simulink model "DYNctl_ver4_etud_Avec_AsservissementNONfonctionnel"  (R2021b)
settings: Solver=ode45  StartTime=0.0  StopTime=tfin  FixedStep=0.001  RelTol=1e-09  EnableMultiTasking=on
values from neighbouring files (symbols this model uses):
  A = num_pos_sph(3)    [Compensateur.m]    (also in matrice_L.m = sym(zeros(13, 13)))
  ae0 = 0.000013398315537 * 1.0e+5    (= 1.3398315537)    [bancEssaiConstantes.m]
  ae1 = 0.003556457401249 * 1.0e+5    (= 355.645740125)    [bancEssaiConstantes.m]
  ae2 = 0.018168930792891 * 1.0e+5    (= 1816.89307929)    [bancEssaiConstantes.m]
  ae3 = 7.043847497815494 * 1.0e+5    (= 704384.749782)    [bancEssaiConstantes.m]
  as0 = 0.0609    [bancEssaiConstantes.m]
  as1 = 18.1233    [bancEssaiConstantes.m]
  as2 = 3.1142e+03    (= 3114.2)    [bancEssaiConstantes.m]
  as3 = -2.3281e+05    (= -232810)    [bancEssaiConstantes.m]
  Axeq = 0    [run_bancessai.m]
  Ayeq = 0    [run_bancessai.m]
  B = [B1 ... (first row only)    [matrice_L.m]
  be1 = 13.029359254409743    (= 13.0293592544)    [bancEssaiConstantes.m]
  C = [Tdef C3 C3 C3 C2 ... (first row only)    [matrice_L.m]
  D = [sum(distance);sum(distance.*voltage)]    [Capteur.m]    (also in matrice_L.m = [0])
  g = 9.81    [bancEssaiConstantes.m]    (also in courant_voltage.m; matrice_L.m; projet.m; trajectoire.m = sqrt(1+(yd).^2))
  Jy = Jx    (= 0.001169)    [bancEssaiConstantes.m]    (also in courant_voltage.m = 0.001347; matrice_L.m = 0.001347)
  Kp_pos_sph = (wn_pos_sph^2)/A_pos_sph    [Compensateur_position_sphere.m]
  Kv_pos_sph = (2*zeta_pos_sph*wn_pos_sph)/A_pos_sph    [Compensateur_position_sphere.m]
  LA = LL    (= 0.115)    [bancEssaiConstantes.m]
  LB = LL    (= 0.115)    [bancEssaiConstantes.m]
  LC = LL    (= 0.115)    [bancEssaiConstantes.m]
  mS = 0.0080    (= 0.008)    [bancEssaiConstantes.m]
  mtot = mP + sig*mS    [bancEssaiConstantes.m]
  Px_eq_simu = double(Px_eq)    [matrice_L.m]
  Py_eq_simu = double(Py_eq)    [matrice_L.m]
  Pzeq = .015    (= 0.015)    [run_bancessai.m]
  RA = RR    (= 3.6)    [bancEssaiConstantes.m]
  RB = RR    (= 3.6)    [bancEssaiConstantes.m]
  RC = RR    (= 3.6)    [bancEssaiConstantes.m]
  TABC_inv = inv(TABC)    [bancEssaiConstantes.m]
  TDEF_inv = inv(TDEF)    [bancEssaiConstantes.m]
  Uinv = inv(U)    [matrice_L.m]
  Va_eq_simu = double(Va_eq)    [courant_voltage.m]
  Vb_eq_simu = double(Vb_eq)    [courant_voltage.m]
  Vc_eq_simu = double(Vc_eq)    [courant_voltage.m]
  Vmax = 22.0    (= 22)    [bancEssaiConstantes.m]
  XB = -rABC*sind(30)    [bancEssaiConstantes.m]    (also in courant_voltage.m = - XA*sind(30); matrice_L.m = -XA*sind(30); projet.m = XA*sind(30))
  XC = -rABC*sind(30)    [bancEssaiConstantes.m]    (also in courant_voltage.m = - XA*sind(30); matrice_L.m = -XA*sind(30); projet.m = XA*sind(30))
  YB = +rABC*cosd(30)    [bancEssaiConstantes.m]    (also in courant_voltage.m = XA*cosd(30); matrice_L.m = XA*cosd(30))
  YC = -rABC*cosd(30)    [bancEssaiConstantes.m]    (also in courant_voltage.m = -XA*cosd(30); matrice_L.m = -XA*cosd(30))
undefined symbols (not defined in the file or in its folder): A_phi, A_s, A_theta, A_z, B_phi, B_sx, B_sy, B_theta, B_z, C_dec, C_s, D_dec, D_s, den_hpc2, den_ip, num_hpc2, num_ip, Tdeft, Tdeft2, U_U_simu
(part 2 of 2)

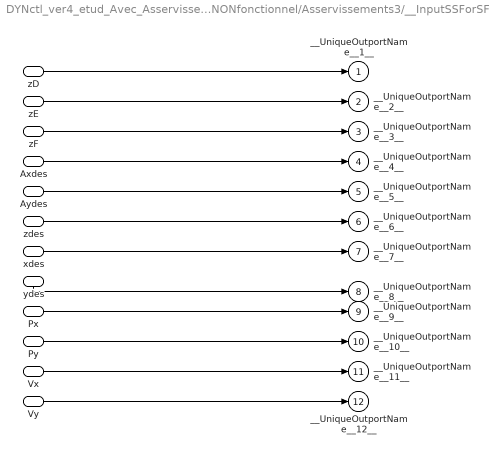
== system DYNctl_ver4_etud_Avec_AsservissementNONfonctionnel/Asservissements3/__InputSSForSFun__ ==
  zD : Inport
  zE : Inport  Port=2
  zF : Inport  Port=3
  Axdes : Inport  Port=4
  Aydes : Inport  Port=5
  zdes : Inport  Port=6
  xdes : Inport  Port=7
  ydes : Inport  Port=8
  Px : Inport  Port=9
  Py : Inport  Port=10
  Vx : Inport  Port=11
  Vy : Inport  Port=12
  __UniqueOutportName__1__ : Outport  VectorParamsAs1DForOutWhenUnconnected=off
  __UniqueOutportName__2__ : Outport  Port=2  VectorParamsAs1DForOutWhenUnconnected=off
  __UniqueOutportName__3__ : Outport  Port=3  VectorParamsAs1DForOutWhenUnconnected=off
  __UniqueOutportName__4__ : Outport  Port=4  VectorParamsAs1DForOutWhenUnconnected=off
  __UniqueOutportName__5__ : Outport  Port=5  VectorParamsAs1DForOutWhenUnconnected=off
  __UniqueOutportName__6__ : Outport  Port=6  VectorParamsAs1DForOutWhenUnconnected=off
  __UniqueOutportName__7__ : Outport  Port=7  VectorParamsAs1DForOutWhenUnconnected=off
  __UniqueOutportName__8__ : Outport  Port=8  VectorParamsAs1DForOutWhenUnconnected=off
  __UniqueOutportName__9__ : Outport  Port=9  VectorParamsAs1DForOutWhenUnconnected=off
  __UniqueOutportName__10__ : Outport  Port=10  VectorParamsAs1DForOutWhenUnconnected=off
  __UniqueOutportName__11__ : Outport  Port=11  VectorParamsAs1DForOutWhenUnconnected=off
  __UniqueOutportName__12__ : Outport  Port=12  VectorParamsAs1DForOutWhenUnconnected=off
  wires:
  zD/1 -> __UniqueOutportName__1__/1
  zE/1 -> __UniqueOutportName__2__/1
  zF/1 -> __UniqueOutportName__3__/1
  Axdes/1 -> __UniqueOutportName__4__/1
  Aydes/1 -> __UniqueOutportName__5__/1
  zdes/1 -> __UniqueOutportName__6__/1
  xdes/1 -> __UniqueOutportName__7__/1
  ydes/1 -> __UniqueOutportName__8__/1
  Px/1 -> __UniqueOutportName__9__/1
  Py/1 -> __UniqueOutportName__10__/1
  Vx/1 -> __UniqueOutportName__11__/1
  Vy/1 -> __UniqueOutportName__12__/1

== system DYNctl_ver4_etud_Avec_AsservissementNONfonctionnel/Asservissements3/__OutputSSForSFun__ ==
  __UniqueInportName__1__ : Inport
  __UniqueInportName__2__ : Inport  Port=2
  __UniqueInportName__3__ : Inport  Port=3
  __UniqueInportName__4__ : Inport  Port=4
  __UniqueInportName__5__ : Inport  Port=5
  VAcalcule : Outport  VectorParamsAs1DForOutWhenUnconnected=off
  VBcalcule : Outport  Port=2  VectorParamsAs1DForOutWhenUnconnected=off
  VCcalcule : Outport  Port=3  VectorParamsAs1DForOutWhenUnconnected=off
  Axcalcule : Outport  Port=4  VectorParamsAs1DForOutWhenUnconnected=off
  Aycalcule : Outport  Port=5  VectorParamsAs1DForOutWhenUnconnected=off
  wires:
  __UniqueInportName__1__/1 -> VAcalcule/1
  __UniqueInportName__2__/1 -> VBcalcule/1
  __UniqueInportName__3__/1 -> VCcalcule/1
  __UniqueInportName__4__/1 -> Axcalcule/1  "Ax_des"
  __UniqueInportName__5__/1 -> Aycalcule/1  "Ay_des"

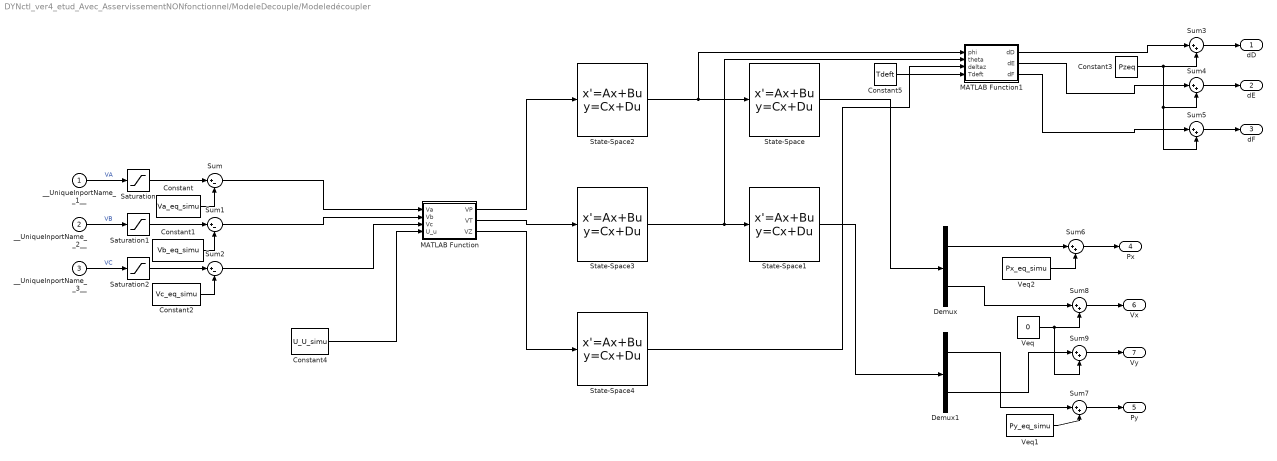
== system DYNctl_ver4_etud_Avec_AsservissementNONfonctionnel/ModeleDecouple/Modeledécoupler ==
  __UniqueInportName__1__ : Inport
  __UniqueInportName__2__ : Inport  Port=2
  __UniqueInportName__3__ : Inport  Port=3
  Constant : Constant  Value=Va_eq_simu
  Constant1 : Constant  Value=Vb_eq_simu
  Constant2 : Constant  Value=Vc_eq_simu
  Constant3 : Constant  Value=Pzeq
  Constant4 : Constant  Value=U_U_simu
  Constant5 : Constant  Value=Tdeft
  Demux : Demux  Outputs=2
  Demux1 : Demux  Outputs=2
  MATLAB Function : MATLAB Function  TreatAsAtomicUnit=on
  MATLAB Function1 : MATLAB Function  TreatAsAtomicUnit=on
  Saturation : Saturate  UpperLimit=Vmax  LowerLimit=-Vmax
  Saturation1 : Saturate  UpperLimit=Vmax  LowerLimit=-Vmax
  Saturation2 : Saturate  UpperLimit=Vmax  LowerLimit=-Vmax
  State-Space : StateSpace  A=A_s  B=B_sx  C=C_s  D=D_s  InitialCondition=0
  State-Space1 : StateSpace  A=A_s  B=B_sy  C=C_s  D=D_s  InitialCondition=0
  State-Space2 : StateSpace  A=A_phi  B=B_phi  C=C_dec  D=D_dec  InitialCondition=0
  State-Space3 : StateSpace  A=A_theta  B=B_theta  C=C_dec  D=D_dec  InitialCondition=0
  State-Space4 : StateSpace  A=A_z  B=B_z  C=C_dec  D=D_dec  InitialCondition=0
  Sum : Sum  Inputs=|+-
  Sum1 : Sum  Inputs=|+-
  Sum2 : Sum  Inputs=|+-
  Sum{3..9} (7 alike) : Sum  Inputs=|++
  Veq : Constant  Value=0  VectorParams1D=off
  Veq1 : Constant  Value=Py_eq_simu
  Veq2 : Constant  Value=Px_eq_simu
  dD : Outport  VectorParamsAs1DForOutWhenUnconnected=off
  dE : Outport  Port=2  VectorParamsAs1DForOutWhenUnconnected=off
  dF : Outport  Port=3  VectorParamsAs1DForOutWhenUnconnected=off
  Px : Outport  Port=4  VectorParamsAs1DForOutWhenUnconnected=off
  Py : Outport  Port=5  VectorParamsAs1DForOutWhenUnconnected=off
  Vx : Outport  Port=6  VectorParamsAs1DForOutWhenUnconnected=off
  Vy : Outport  Port=7  VectorParamsAs1DForOutWhenUnconnected=off
  wires:
  __UniqueInportName__1__/1 -> Saturation/1  "VA"
  __UniqueInportName__2__/1 -> Saturation1/1  "VB"
  __UniqueInportName__3__/1 -> Saturation2/1  "VC"
  Constant/1 -> Sum/2
  Sum/1 -> MATLAB Function/1(Va)
  Constant1/1 -> Sum1/2
  Sum1/1 -> MATLAB Function/2(Vb)
  Constant2/1 -> Sum2/2
  Sum2/1 -> MATLAB Function/3(Vc)
  Sum6/1 -> Px/1
  Sum7/1 -> Py/1
  Sum8/1 -> Vx/1
  Sum9/1 -> Vy/1
  Veq/1 -> Sum8/2, Sum9/2
  Veq1/1 -> Sum7/2
  Veq2/1 -> Sum6/2
  Sum3/1 -> dD/1
  Saturation/1 -> Sum/1
  Saturation1/1 -> Sum1/1
  Saturation2/1 -> Sum2/1
  State-Space3/1 -> MATLAB Function1/2(theta), State-Space1/1
  State-Space2/1 -> MATLAB Function1/1(phi), State-Space/1
  Constant4/1 -> MATLAB Function/4(U_u)
  MATLAB Function/1(VP) -> State-Space2/1
  MATLAB Function/2(VT) -> State-Space3/1
  MATLAB Function/3(VZ) -> State-Space4/1
  State-Space/1 -> Demux/1
  State-Space1/1 -> Demux1/1
  Constant3/1 -> Sum4/2, Sum5/2, Sum3/2
  Sum5/1 -> dF/1
  Sum4/1 -> dE/1
  State-Space4/1 -> MATLAB Function1/3(deltaz)
  Constant5/1 -> MATLAB Function1/4(Tdeft)
  MATLAB Function1/1(dD) -> Sum3/1
  MATLAB Function1/2(dE) -> Sum4/1
  MATLAB Function1/3(dF) -> Sum5/1
  Demux/1 -> Sum6/1
  Demux/2 -> Sum8/1
  Demux1/1 -> Sum7/1
  Demux1/2 -> Sum9/1

== system DYNctl_ver4_etud_Avec_AsservissementNONfonctionnel/ModeleDecouple/__InputSSForSFun__ ==
  VAdesire : Inport
  VBdesire : Inport  Port=2
  VCdesire : Inport  Port=3
  __UniqueOutportName__1__ : Outport  VectorParamsAs1DForOutWhenUnconnected=off
  __UniqueOutportName__2__ : Outport  Port=2  VectorParamsAs1DForOutWhenUnconnected=off
  __UniqueOutportName__3__ : Outport  Port=3  VectorParamsAs1DForOutWhenUnconnected=off
  wires:
  VAdesire/1 -> __UniqueOutportName__1__/1
  VBdesire/1 -> __UniqueOutportName__2__/1
  VCdesire/1 -> __UniqueOutportName__3__/1

== system DYNctl_ver4_etud_Avec_AsservissementNONfonctionnel/ModeleDecouple/__OutputSSForSFun__ ==
  __UniqueInportName__17__1 : Inport
  __UniqueInportName__18__ : Inport  Port=2
  __UniqueInportName__19__ : Inport  Port=3
  __UniqueInportName__7__ : Inport  Port=4
  __UniqueInportName__8__ : Inport  Port=5
  __UniqueInportName__9__ : Inport  Port=6
  __UniqueInportName__10__ : Inport  Port=7
  zD1 : Outport  VectorParamsAs1DForOutWhenUnconnected=off
  zE1 : Outport  Port=2  VectorParamsAs1DForOutWhenUnconnected=off
  zF1 : Outport  Port=3  VectorParamsAs1DForOutWhenUnconnected=off
  Px : Outport  Port=4  VectorParamsAs1DForOutWhenUnconnected=off
  Py : Outport  Port=5  VectorParamsAs1DForOutWhenUnconnected=off
  Vx : Outport  Port=6  VectorParamsAs1DForOutWhenUnconnected=off
  Vy : Outport  Port=7  VectorParamsAs1DForOutWhenUnconnected=off
  wires:
  __UniqueInportName__19__/1 -> zF1/1  "zf"
  __UniqueInportName__18__/1 -> zE1/1  "ze"
  __UniqueInportName__17__1/1 -> zD1/1  "zd"
  __UniqueInportName__10__/1 -> Vy/1  "Vy"
  __UniqueInportName__9__/1 -> Vx/1  "Vx"
  __UniqueInportName__8__/1 -> Py/1  "Py"
  __UniqueInportName__7__/1 -> Px/1  "Px"

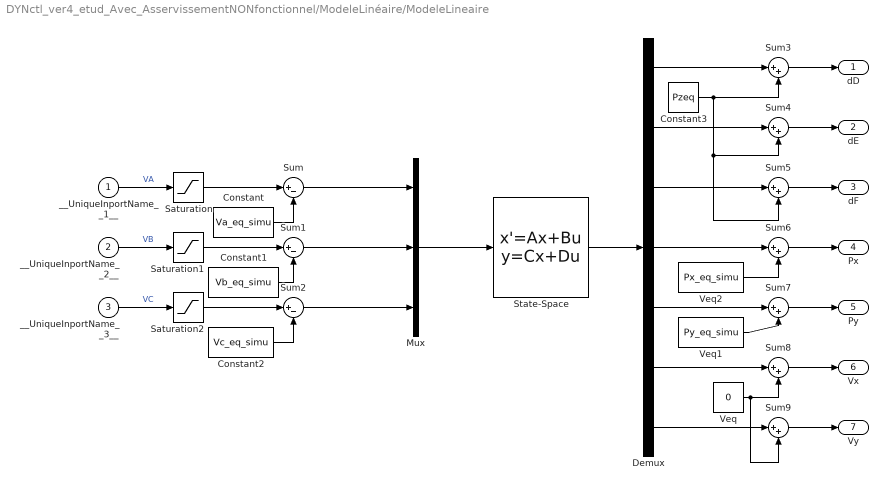
== system DYNctl_ver4_etud_Avec_AsservissementNONfonctionnel/ModeleLinéaire/ModeleLineaire ==
  __UniqueInportName__1__ : Inport
  __UniqueInportName__2__ : Inport  Port=2
  __UniqueInportName__3__ : Inport  Port=3
  Constant : Constant  Value=Va_eq_simu
  Constant1 : Constant  Value=Vb_eq_simu
  Constant2 : Constant  Value=Vc_eq_simu
  Constant3 : Constant  Value=Pzeq
  Demux : Demux  Outputs=7
  Mux : Mux  Inputs=3
  Saturation : Saturate  UpperLimit=Vmax  LowerLimit=-Vmax
  Saturation1 : Saturate  UpperLimit=Vmax  LowerLimit=-Vmax
  Saturation2 : Saturate  UpperLimit=Vmax  LowerLimit=-Vmax
  State-Space : StateSpace  A=A  B=B  C=C  D=D  InitialCondition=0
  Sum : Sum  Inputs=|+-
  Sum1 : Sum  Inputs=|+-
  Sum2 : Sum  Inputs=|+-
  Sum{3..9} (7 alike) : Sum  Inputs=|++
  Veq : Constant  Value=0
  Veq1 : Constant  Value=Py_eq_simu
  Veq2 : Constant  Value=Px_eq_simu
  dD : Outport  VectorParamsAs1DForOutWhenUnconnected=off
  dE : Outport  Port=2  VectorParamsAs1DForOutWhenUnconnected=off
  dF : Outport  Port=3  VectorParamsAs1DForOutWhenUnconnected=off
  Px : Outport  Port=4  VectorParamsAs1DForOutWhenUnconnected=off
  Py : Outport  Port=5  VectorParamsAs1DForOutWhenUnconnected=off
  Vx : Outport  Port=6  VectorParamsAs1DForOutWhenUnconnected=off
  Vy : Outport  Port=7  VectorParamsAs1DForOutWhenUnconnected=off
  wires:
  __UniqueInportName__1__/1 -> Saturation/1  "VA"
  __UniqueInportName__2__/1 -> Saturation1/1  "VB"
  __UniqueInportName__3__/1 -> Saturation2/1  "VC"
  Mux/1 -> State-Space/1
  State-Space/1 -> Demux/1
  Constant/1 -> Sum/2
  Sum/1 -> Mux/1
  Constant1/1 -> Sum1/2
  Sum1/1 -> Mux/2
  Constant2/1 -> Sum2/2
  Sum2/1 -> Mux/3
  Sum6/1 -> Px/1
  Sum7/1 -> Py/1
  Sum8/1 -> Vx/1
  Sum9/1 -> Vy/1
  Veq/1 -> Sum9/2, Sum8/2
  Demux/7 -> Sum9/1
  Demux/6 -> Sum8/1
  Veq1/1 -> Sum7/2
  Demux/5 -> Sum7/1
  Veq2/1 -> Sum6/2
  Demux/4 -> Sum6/1
  Constant3/1 -> Sum3/2, Sum4/2, Sum5/2
  Demux/1 -> Sum3/1
  Demux/2 -> Sum4/1
  Demux/3 -> Sum5/1
  Sum5/1 -> dF/1
  Sum3/1 -> dD/1
  Sum4/1 -> dE/1
  Saturation/1 -> Sum/1
  Saturation1/1 -> Sum1/1
  Saturation2/1 -> Sum2/1

== system DYNctl_ver4_etud_Avec_AsservissementNONfonctionnel/ModeleLinéaire/__InputSSForSFun__ ==
  VAdesire : Inport
  VBdesire : Inport  Port=2
  VCdesire : Inport  Port=3
  __UniqueOutportName__1__ : Outport  VectorParamsAs1DForOutWhenUnconnected=off
  __UniqueOutportName__2__ : Outport  Port=2  VectorParamsAs1DForOutWhenUnconnected=off
  __UniqueOutportName__3__ : Outport  Port=3  VectorParamsAs1DForOutWhenUnconnected=off
  wires:
  VAdesire/1 -> __UniqueOutportName__1__/1
  VBdesire/1 -> __UniqueOutportName__2__/1
  VCdesire/1 -> __UniqueOutportName__3__/1

== system DYNctl_ver4_etud_Avec_AsservissementNONfonctionnel/ModeleLinéaire/__OutputSSForSFun__ ==
  __UniqueInportName__17__ : Inport
  __UniqueInportName__18__ : Inport  Port=2
  __UniqueInportName__19__ : Inport  Port=3
  __UniqueInportName__7__ : Inport  Port=4
  __UniqueInportName__8__ : Inport  Port=5
  __UniqueInportName__9__ : Inport  Port=6
  __UniqueInportName__10__ : Inport  Port=7
  zD : Outport  VectorParamsAs1DForOutWhenUnconnected=off
  zE : Outport  Port=2  VectorParamsAs1DForOutWhenUnconnected=off
  zF : Outport  Port=3  VectorParamsAs1DForOutWhenUnconnected=off
  Px : Outport  Port=4  VectorParamsAs1DForOutWhenUnconnected=off
  Py : Outport  Port=5  VectorParamsAs1DForOutWhenUnconnected=off
  Vx : Outport  Port=6  VectorParamsAs1DForOutWhenUnconnected=off
  Vy : Outport  Port=7  VectorParamsAs1DForOutWhenUnconnected=off
  wires:
  __UniqueInportName__7__/1 -> Px/1  "Px"
  __UniqueInportName__8__/1 -> Py/1  "Py"
  __UniqueInportName__9__/1 -> Vx/1  "Vx"
  __UniqueInportName__10__/1 -> Vy/1  "Vy"
  __UniqueInportName__17__/1 -> zD/1  "zd"
  __UniqueInportName__18__/1 -> zE/1  "ze"
  __UniqueInportName__19__/1 -> zF/1  "zf"

== system DYNctl_ver4_etud_Avec_AsservissementNONfonctionnel/ModeleNonLineaire/__InputSSForSFun__ ==
  VAdesire : Inport
  VBdesire : Inport  Port=2
  VCdesire : Inport  Port=3
  __UniqueOutportName__1__ : Outport
  __UniqueOutportName__2__ : Outport  Port=2
  __UniqueOutportName__3__ : Outport  Port=3
  wires:
  VAdesire/1 -> __UniqueOutportName__1__/1
  VBdesire/1 -> __UniqueOutportName__2__/1
  VCdesire/1 -> __UniqueOutportName__3__/1

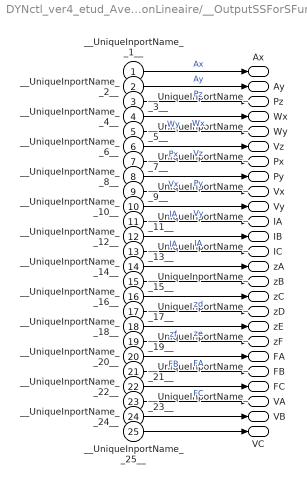
== system DYNctl_ver4_etud_Avec_AsservissementNONfonctionnel/ModeleNonLineaire/__OutputSSForSFun__ ==
  __UniqueInportName__1__ : Inport
  __UniqueInportName__2__ : Inport  Port=2
  __UniqueInportName__3__ : Inport  Port=3
  __UniqueInportName__4__ : Inport  Port=4
  __UniqueInportName__5__ : Inport  Port=5
  __UniqueInportName__6__ : Inport  Port=6
  __UniqueInportName__7__ : Inport  Port=7
  __UniqueInportName__8__ : Inport  Port=8
  __UniqueInportName__9__ : Inport  Port=9
  __UniqueInportName__10__ : Inport  Port=10
  __UniqueInportName__11__ : Inport  Port=11
  __UniqueInportName__12__ : Inport  Port=12
  __UniqueInportName__13__ : Inport  Port=13
  __UniqueInportName__14__ : Inport  Port=14
  __UniqueInportName__15__ : Inport  Port=15
  __UniqueInportName__16__ : Inport  Port=16
  __UniqueInportName__17__ : Inport  Port=17
  __UniqueInportName__18__ : Inport  Port=18
  __UniqueInportName__19__ : Inport  Port=19
  __UniqueInportName__20__ : Inport  Port=20
  __UniqueInportName__21__ : Inport  Port=21
  __UniqueInportName__22__ : Inport  Port=22
  __UniqueInportName__23__ : Inport  Port=23
  __UniqueInportName__24__ : Inport  Port=24
  __UniqueInportName__25__ : Inport  Port=25
  Ax : Outport
  Ay : Outport  Port=2
  Pz : Outport  Port=3
  Wx : Outport  Port=4
  Wy : Outport  Port=5
  Vz : Outport  Port=6
  Px : Outport  Port=7
  Py : Outport  Port=8
  Vx : Outport  Port=9
  Vy : Outport  Port=10
  IA : Outport  Port=11
  IB : Outport  Port=12
  IC : Outport  Port=13
  zA : Outport  Port=14
  zB : Outport  Port=15
  zC : Outport  Port=16
  zD : Outport  Port=17
  zE : Outport  Port=18
  zF : Outport  Port=19
  FA : Outport  Port=20
  FB : Outport  Port=21
  FC : Outport  Port=22
  VA : Outport  Port=23
  VB : Outport  Port=24
  VC : Outport  Port=25
  wires:
  __UniqueInportName__1__/1 -> Ax/1  "Ax"
  __UniqueInportName__2__/1 -> Ay/1  "Ay"
  __UniqueInportName__3__/1 -> Pz/1  "Pz"
  __UniqueInportName__4__/1 -> Wx/1  "Wx"
  __UniqueInportName__5__/1 -> Wy/1  "Wy"
  __UniqueInportName__6__/1 -> Vz/1  "Vz"
  __UniqueInportName__7__/1 -> Px/1  "Px"
  __UniqueInportName__8__/1 -> Py/1  "Py"
  __UniqueInportName__9__/1 -> Vx/1  "Vx"
  __UniqueInportName__10__/1 -> Vy/1  "Vy"
  __UniqueInportName__11__/1 -> IA/1  "IA"
  __UniqueInportName__12__/1 -> IB/1  "IA"
  __UniqueInportName__13__/1 -> IC/1  "IA"
  __UniqueInportName__14__/1 -> zA/1
  __UniqueInportName__15__/1 -> zB/1
  __UniqueInportName__16__/1 -> zC/1
  __UniqueInportName__17__/1 -> zD/1  "zd"
  __UniqueInportName__18__/1 -> zE/1  "ze"
  __UniqueInportName__19__/1 -> zF/1  "zf"
  __UniqueInportName__20__/1 -> FA/1  "FA"
  __UniqueInportName__21__/1 -> FB/1  "FB"
  __UniqueInportName__22__/1 -> FC/1  "FC"
  __UniqueInportName__23__/1 -> VA/1
  __UniqueInportName__24__/1 -> VB/1
  __UniqueInportName__25__/1 -> VC/1

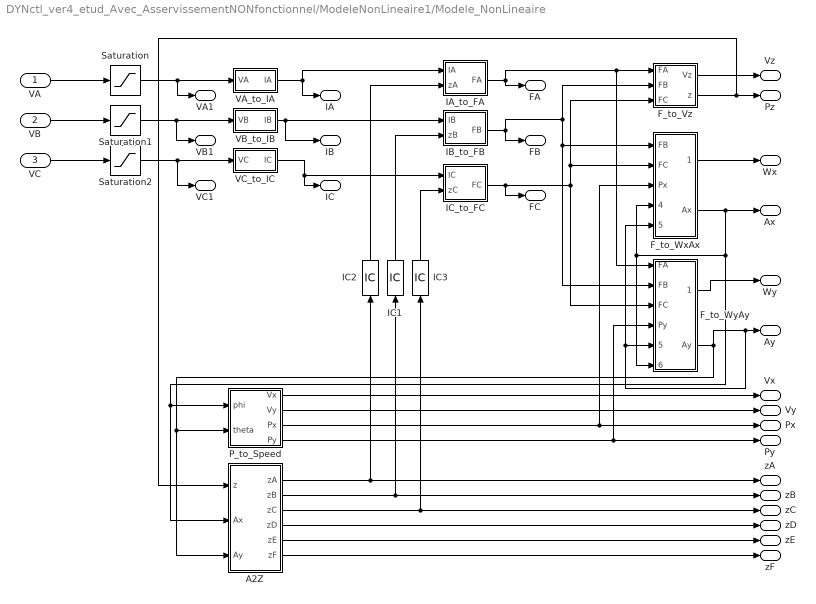
== system DYNctl_ver4_etud_Avec_AsservissementNONfonctionnel/ModeleNonLineaire1/Modele_NonLineaire ==
  VA : Inport
  VB : Inport  Port=2
  VC : Inport  Port=3
  A2Z : Subsystem
  F_to_Vz : Subsystem
  F_to_WxAx : Subsystem
  F_to_WyAy : Subsystem
  IA_to_FA : Subsystem
  IB_to_FB : Subsystem
  IC1 : InitialCondition  Value=Pzeq
  IC2 : InitialCondition  Value=Pzeq
  IC3 : InitialCondition  Value=Pzeq
  IC_to_FC : Subsystem
  P_to_Speed : Subsystem
  Saturation : Saturate  UpperLimit=Vmax  LowerLimit=-Vmax
  Saturation1 : Saturate  UpperLimit=Vmax  LowerLimit=-Vmax
  Saturation2 : Saturate  UpperLimit=Vmax  LowerLimit=-Vmax
  VA_to_IA : Subsystem
  VB_to_IB : Subsystem
  VC_to_IC : Subsystem
  Ax : Outport
  Ay : Outport  Port=2
  Pz : Outport  Port=3
  Wx : Outport  Port=4
  Wy : Outport  Port=5
  Vz : Outport  Port=6
  Px : Outport  Port=7
  Py : Outport  Port=8
  Vx : Outport  Port=9
  Vy : Outport  Port=10
  IA : Outport  Port=11
  IB : Outport  Port=12
  IC : Outport  Port=13
  zA : Outport  Port=14
  zB : Outport  Port=15
  zC : Outport  Port=16
  zD : Outport  Port=17
  zE : Outport  Port=18
  zF : Outport  Port=19
  FA : Outport  Port=20
  FB : Outport  Port=21
  FC : Outport  Port=22
  VA1 : Outport  Port=23
  VB1 : Outport  Port=24
  VC1 : Outport  Port=25
  wires:
  VA/1 -> Saturation/1
  VB/1 -> Saturation1/1
  VC/1 -> Saturation2/1
  VA_to_IA/1(IA) -> IA/1, IA_to_FA/1(IA)
  VB_to_IB/1(IB) -> IB/1, IB_to_FB/1(IB)
  VC_to_IC/1(IC) -> IC_to_FC/1(IC), IC/1
  IC_to_FC/1(FC) -> F_to_WyAy/3(FC), F_to_WxAx/2(FC), F_to_Vz/3(FC), FC/1
  IB_to_FB/1(FB) -> F_to_WyAy/2(FB), F_to_WxAx/1(FB), F_to_Vz/2(FB), FB/1
  IA_to_FA/1(FA) -> F_to_WyAy/1(FA), F_to_Vz/1(FA), FA/1
  F_to_WxAx/2(Ax) -> P_to_Speed/1(phi), A2Z/2(Ax), F_to_WyAy/6(phi), F_to_WxAx/4(phi), Ax/1
  F_to_WyAy/2(Ay) -> F_to_WxAx/5(theta), F_to_WyAy/5(theta), Ay/1, P_to_Speed/2(theta), A2Z/3(Ay)
  F_to_WyAy/1(Wy) -> Wy/1
  F_to_Vz/1(Vz) -> Vz/1
  F_to_WxAx/1(Wx) -> Wx/1
  P_to_Speed/1(Vx) -> Vx/1
  P_to_Speed/2(Vy) -> Vy/1
  F_to_Vz/2(z) -> A2Z/1(z), Pz/1
  P_to_Speed/3(Px) -> Px/1, F_to_WxAx/3(Px)
  P_to_Speed/4(Py) -> Py/1, F_to_WyAy/4(Py)
  A2Z/6(zF) -> zF/1
  A2Z/1(zA) -> zA/1, IC2/1
  A2Z/5(zE) -> zE/1
  A2Z/2(zB) -> zB/1, IC1/1
  A2Z/3(zC) -> zC/1, IC3/1
  A2Z/4(zD) -> zD/1
  Saturation/1 -> VA1/1, VA_to_IA/1(VA)
  Saturation1/1 -> VB1/1, VB_to_IB/1(VB)
  Saturation2/1 -> VC1/1, VC_to_IC/1(VC)
  IC2/1 -> IA_to_FA/2(zA)
  IC1/1 -> IB_to_FB/2(zB)
  IC3/1 -> IC_to_FC/2(zC)

== system DYNctl_ver4_etud_Avec_AsservissementNONfonctionnel/ModeleNonLineaire1/__InputSSForSFun__ ==
  VAdesire : Inport
  VBdesire : Inport  Port=2
  VCdesire : Inport  Port=3
  __UniqueOutportName__1__ : Outport
  __UniqueOutportName__2__ : Outport  Port=2
  __UniqueOutportName__3__ : Outport  Port=3
  wires:
  VAdesire/1 -> __UniqueOutportName__1__/1
  VBdesire/1 -> __UniqueOutportName__2__/1
  VCdesire/1 -> __UniqueOutportName__3__/1

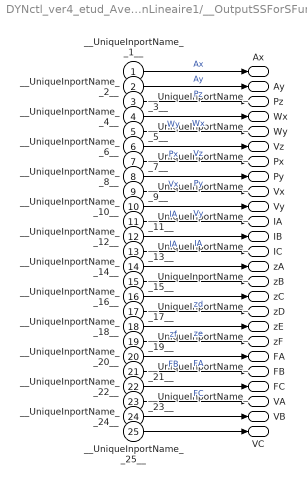
== system DYNctl_ver4_etud_Avec_AsservissementNONfonctionnel/ModeleNonLineaire1/__OutputSSForSFun__ ==
  __UniqueInportName__1__ : Inport
  __UniqueInportName__2__ : Inport  Port=2
  __UniqueInportName__3__ : Inport  Port=3
  __UniqueInportName__4__ : Inport  Port=4
  __UniqueInportName__5__ : Inport  Port=5
  __UniqueInportName__6__ : Inport  Port=6
  __UniqueInportName__7__ : Inport  Port=7
  __UniqueInportName__8__ : Inport  Port=8
  __UniqueInportName__9__ : Inport  Port=9
  __UniqueInportName__10__ : Inport  Port=10
  __UniqueInportName__11__ : Inport  Port=11
  __UniqueInportName__12__ : Inport  Port=12
  __UniqueInportName__13__ : Inport  Port=13
  __UniqueInportName__14__ : Inport  Port=14
  __UniqueInportName__15__ : Inport  Port=15
  __UniqueInportName__16__ : Inport  Port=16
  __UniqueInportName__17__ : Inport  Port=17
  __UniqueInportName__18__ : Inport  Port=18
  __UniqueInportName__19__ : Inport  Port=19
  __UniqueInportName__20__ : Inport  Port=20
  __UniqueInportName__21__ : Inport  Port=21
  __UniqueInportName__22__ : Inport  Port=22
  __UniqueInportName__23__ : Inport  Port=23
  __UniqueInportName__24__ : Inport  Port=24
  __UniqueInportName__25__ : Inport  Port=25
  Ax : Outport
  Ay : Outport  Port=2
  Pz : Outport  Port=3
  Wx : Outport  Port=4
  Wy : Outport  Port=5
  Vz : Outport  Port=6
  Px : Outport  Port=7
  Py : Outport  Port=8
  Vx : Outport  Port=9
  Vy : Outport  Port=10
  IA : Outport  Port=11
  IB : Outport  Port=12
  IC : Outport  Port=13
  zA : Outport  Port=14
  zB : Outport  Port=15
  zC : Outport  Port=16
  zD : Outport  Port=17
  zE : Outport  Port=18
  zF : Outport  Port=19
  FA : Outport  Port=20
  FB : Outport  Port=21
  FC : Outport  Port=22
  VA : Outport  Port=23
  VB : Outport  Port=24
  VC : Outport  Port=25
  wires:
  __UniqueInportName__1__/1 -> Ax/1  "Ax"
  __UniqueInportName__2__/1 -> Ay/1  "Ay"
  __UniqueInportName__3__/1 -> Pz/1  "Pz"
  __UniqueInportName__4__/1 -> Wx/1  "Wx"
  __UniqueInportName__5__/1 -> Wy/1  "Wy"
  __UniqueInportName__6__/1 -> Vz/1  "Vz"
  __UniqueInportName__7__/1 -> Px/1  "Px"
  __UniqueInportName__8__/1 -> Py/1  "Py"
  __UniqueInportName__9__/1 -> Vx/1  "Vx"
  __UniqueInportName__10__/1 -> Vy/1  "Vy"
  __UniqueInportName__11__/1 -> IA/1  "IA"
  __UniqueInportName__12__/1 -> IB/1  "IA"
  __UniqueInportName__13__/1 -> IC/1  "IA"
  __UniqueInportName__14__/1 -> zA/1
  __UniqueInportName__15__/1 -> zB/1
  __UniqueInportName__16__/1 -> zC/1
  __UniqueInportName__17__/1 -> zD/1  "zd"
  __UniqueInportName__18__/1 -> zE/1  "ze"
  __UniqueInportName__19__/1 -> zF/1  "zf"
  __UniqueInportName__20__/1 -> FA/1  "FA"
  __UniqueInportName__21__/1 -> FB/1  "FB"
  __UniqueInportName__22__/1 -> FC/1  "FC"
  __UniqueInportName__23__/1 -> VA/1
  __UniqueInportName__24__/1 -> VB/1
  __UniqueInportName__25__/1 -> VC/1

== system DYNctl_ver4_etud_Avec_AsservissementNONfonctionnel/ModeleNonLineaire1/Modele_NonLineaire/A2Z ==
  z : Inport
  Ax : Inport  Port=2
  Ay : Inport  Port=3
  IC : InitialCondition  Value=Pzeq
  IC1 : InitialCondition  Value=Ayeq
  IC2 : InitialCondition  Value=Axeq
  MATLAB Function : MATLAB Function  TreatAsAtomicUnit=on
  zA : Outport  VectorParamsAs1DForOutWhenUnconnected=off
  zB : Outport  Port=2  VectorParamsAs1DForOutWhenUnconnected=off
  zC : Outport  Port=3  VectorParamsAs1DForOutWhenUnconnected=off
  zD : Outport  Port=4  VectorParamsAs1DForOutWhenUnconnected=off
  zE : Outport  Port=5  VectorParamsAs1DForOutWhenUnconnected=off
  zF : Outport  Port=6  VectorParamsAs1DForOutWhenUnconnected=off
  wires:
  z/1 -> IC/1
  Ay/1 -> IC1/1
  Ax/1 -> IC2/1
  IC/1 -> MATLAB Function/1(z)
  IC1/1 -> MATLAB Function/2(Ax)
  IC2/1 -> MATLAB Function/3(Ay)
  MATLAB Function/6(zF) -> zF/1
  MATLAB Function/5(zE) -> zE/1
  MATLAB Function/4(zD) -> zD/1
  MATLAB Function/1(zA) -> zA/1
  MATLAB Function/2(zB) -> zB/1
  MATLAB Function/3(zC) -> zC/1

== system DYNctl_ver4_etud_Avec_AsservissementNONfonctionnel/ModeleNonLineaire1/Modele_NonLineaire/F_to_Vz ==
  FA : Inport
  FB : Inport  Port=2
  FC : Inport  Port=3
  Integrator : Integrator
  Integrator1 : Integrator  InitialCondition=Pzeq
  MATLAB Function : MATLAB Function  TreatAsAtomicUnit=on
  Vz : Outport  VectorParamsAs1DForOutWhenUnconnected=off
  z : Outport  Port=2  VectorParamsAs1DForOutWhenUnconnected=off
  wires:
  MATLAB Function/1(d2z) -> Integrator/1
  Integrator/1 -> Integrator1/1, Vz/1
  Integrator1/1 -> z/1
  FA/1 -> MATLAB Function/1(FA)
  FB/1 -> MATLAB Function/2(FB)
  FC/1 -> MATLAB Function/3(FC)

== system DYNctl_ver4_etud_Avec_AsservissementNONfonctionnel/ModeleNonLineaire1/Modele_NonLineaire/F_to_WxAx ==
  FB : Inport
  FC : Inport  Port=2
  Px : Inport  Port=3
  phi : Inport  Port=4
  theta : Inport  Port=5
  Integrator : Integrator
  Integrator1 : Integrator
  MATLAB Function : MATLAB Function  TreatAsAtomicUnit=on
  Wx : Outport  VectorParamsAs1DForOutWhenUnconnected=off
  Ax : Outport  Port=2  VectorParamsAs1DForOutWhenUnconnected=off
  wires:
  Integrator/1 -> Integrator1/1, Wx/1
  Integrator1/1 -> Ax/1
  FB/1 -> MATLAB Function/1(FB)
  FC/1 -> MATLAB Function/2(FC)
  Px/1 -> MATLAB Function/3(Py)
  phi/1 -> MATLAB Function/4(Ax)
  theta/1 -> ?
  MATLAB Function/1(d2phi) -> Integrator/1

== system DYNctl_ver4_etud_Avec_AsservissementNONfonctionnel/ModeleNonLineaire1/Modele_NonLineaire/F_to_WyAy ==
  FA : Inport
  FB : Inport  Port=2
  FC : Inport  Port=3
  Py : Inport  Port=4
  theta : Inport  Port=5
  phi : Inport  Port=6
  Integrator : Integrator
  Integrator1 : Integrator
  MATLAB Function : MATLAB Function  TreatAsAtomicUnit=on
  Wy : Outport  VectorParamsAs1DForOutWhenUnconnected=off
  Ay : Outport  Port=2  VectorParamsAs1DForOutWhenUnconnected=off
  wires:
  FB/1 -> MATLAB Function/2(FB)
  FC/1 -> MATLAB Function/3(FC)
  Integrator/1 -> Integrator1/1, Wy/1
  Integrator1/1 -> Ay/1
  Py/1 -> MATLAB Function/6(Py)
  FA/1 -> MATLAB Function/1(FA)
  theta/1 -> MATLAB Function/4(phi)
  phi/1 -> MATLAB Function/5(theta)
  MATLAB Function/1(d2theta) -> Integrator/1

== system DYNctl_ver4_etud_Avec_AsservissementNONfonctionnel/ModeleNonLineaire1/Modele_NonLineaire/IA_to_FA ==
  IA : Inport
  zA : Inport  Port=2
  MATLAB Function : MATLAB Function  TreatAsAtomicUnit=on
  FA : Outport  VectorParamsAs1DForOutWhenUnconnected=off
  wires:
  MATLAB Function/1(F) -> FA/1
  IA/1 -> MATLAB Function/1(I)
  zA/1 -> MATLAB Function/2(Z)

== system DYNctl_ver4_etud_Avec_AsservissementNONfonctionnel/ModeleNonLineaire1/Modele_NonLineaire/IB_to_FB ==
  IB : Inport
  zB : Inport  Port=2
  MATLAB Function : MATLAB Function  TreatAsAtomicUnit=on
  FB : Outport  VectorParamsAs1DForOutWhenUnconnected=off
  wires:
  zB/1 -> MATLAB Function/2(Z)
  MATLAB Function/1(F) -> FB/1
  IB/1 -> MATLAB Function/1(I)

== system DYNctl_ver4_etud_Avec_AsservissementNONfonctionnel/ModeleNonLineaire1/Modele_NonLineaire/IC_to_FC ==
  IC : Inport
  zC : Inport  Port=2
  MATLAB Function : MATLAB Function  TreatAsAtomicUnit=on
  FC : Outport  VectorParamsAs1DForOutWhenUnconnected=off
  wires:
  zC/1 -> MATLAB Function/2(Z)
  MATLAB Function/1(F) -> FC/1
  IC/1 -> MATLAB Function/1(I)

== system DYNctl_ver4_etud_Avec_AsservissementNONfonctionnel/ModeleNonLineaire1/Modele_NonLineaire/P_to_Speed ==
  phi : Inport
  theta : Inport  Port=2
  Gain : Gain  Gain=-5*g/7
  Gain1 : Gain  Gain=5*g/7
  Integrator{,1..3} (4 alike) : Integrator
  Vx : Outport
  Vy : Outport  Port=2
  Px : Outport  Port=3
  Py : Outport  Port=4
  wires:
  theta/1 -> Gain1/1
  phi/1 -> Gain/1
  Gain/1 -> Integrator/1
  Gain1/1 -> Integrator1/1
  Integrator/1 -> Integrator2/1, Vx/1
  Integrator1/1 -> Integrator3/1, Vy/1
  Integrator2/1 -> Px/1
  Integrator3/1 -> Py/1

== system DYNctl_ver4_etud_Avec_AsservissementNONfonctionnel/ModeleNonLineaire1/Modele_NonLineaire/VA_to_IA ==
  VA : Inport
  Gain : Gain  Gain=1/LA
  Gain1 : Gain  Gain=RA/LA
  Integrator : Integrator  InitialCondition=-0.496058088227384
  Subtract : Sum  Inputs=+-
  IA : Outport  VectorParamsAs1DForOutWhenUnconnected=off
  wires:
  VA/1 -> Gain/1
  Integrator/1 -> IA/1, Gain1/1
  Subtract/1 -> Integrator/1
  Gain/1 -> Subtract/1
  Gain1/1 -> Subtract/2

== system DYNctl_ver4_etud_Avec_AsservissementNONfonctionnel/ModeleNonLineaire1/Modele_NonLineaire/VB_to_IB ==
  VB : Inport
  Gain : Gain  Gain=1/LB
  Gain1 : Gain  Gain=RB/LB
  Integrator : Integrator  InitialCondition=-0.496058088227384
  Subtract : Sum  Inputs=+-
  IB : Outport  VectorParamsAs1DForOutWhenUnconnected=off
  wires:
  VB/1 -> Gain/1
  Integrator/1 -> IB/1, Gain1/1
  Subtract/1 -> Integrator/1
  Gain/1 -> Subtract/1
  Gain1/1 -> Subtract/2

== system DYNctl_ver4_etud_Avec_AsservissementNONfonctionnel/ModeleNonLineaire1/Modele_NonLineaire/VC_to_IC ==
  VC : Inport
  Gain : Gain  Gain=1/LC
  Gain1 : Gain  Gain=RC/LC
  Integrator : Integrator  InitialCondition=-0.496058088227384
  Subtract : Sum  Inputs=+-
  IC : Outport  VectorParamsAs1DForOutWhenUnconnected=off
  wires:
  VC/1 -> Gain/1
  Integrator/1 -> IC/1, Gain1/1
  Subtract/1 -> Integrator/1
  Gain/1 -> Subtract/1
  Gain1/1 -> Subtract/2

== matlab function DYNctl_ver4_etud_Avec_AsservissementNONfonctionnel/ModeleNonLineaire1/Modele_NonLineaire/F_to_WyAy/MATLAB Function ==
  data: FA input; FB input; FC input; phi input; theta input; g parameter; d2theta output; XB parameter; mS parameter; XC parameter; Jy parameter; Py input
function d2theta = fcn(FA,FB,FC,phi,theta,g,XB,mS, XC, Jy, Py)

d2theta = 0;

== matlab function DYNctl_ver4_etud_Avec_AsservissementNONfonctionnel/ModeleNonLineaire1/Modele_NonLineaire/A2Z/MATLAB Function ==
  data: z input; Ax input; Ay input; zA output; zB output; zC output; zD output; zE output; zF output; TABC_inv parameter; TDEF_inv parameter
function [zA,zB,zC,zD,zE,zF] = fcn(z,Ax,Ay,TABC_inv, TDEF_inv)

u = [Ax;Ay;z];

zA = TABC_inv(1,:)*u;
zB = TABC_inv(2,:)*u;
zC = TABC_inv(3,:)*u;
zD = TDEF_inv(1,:)*u;
zE = TDEF_inv(2,:)*u;
zF = TDEF_inv(3,:)*u;

== matlab function DYNctl_ver4_etud_Avec_AsservissementNONfonctionnel/ModeleDecouple/Modeledécoupler/MATLAB Function ==
  data: Va input; VP output; Vb input; Vc input; U_u input; VT output; VZ output
function [VP,VT,VZ] = fcn(Va, Vb, Vc,U_u)

V = U_u*[Va Vb Vc]';
VP = V(1);
VT = V(2);
VZ = V(3);

== matlab function DYNctl_ver4_etud_Avec_AsservissementNONfonctionnel/ModeleDecouple/Modeledécoupler/MATLAB Function1 ==
  data: phi input; dD output; theta input; deltaz input; Tdeft input; dE output; dF output
function [dD,dE,dF] = fcn(phi, theta, deltaz,Tdeft)

Yp = Tdeft*[phi theta deltaz]';
dD = Yp(1);
dE = Yp(2);
dF = Yp(3);

== matlab function DYNctl_ver4_etud_Avec_AsservissementNONfonctionnel/ModeleNonLineaire1/Modele_NonLineaire/IB_to_FB/MATLAB Function ==
  data: I input; F output; Z input; ae0 parameter; ae1 parameter; ae2 parameter; ae3 parameter; as0 parameter; as1 parameter; as2 parameter; as3 parameter; be1 parameter
function F = fcn(I,Z,ae0, ae1, ae2, ae3, as0, as1, as2, as3,be1)

F = ((I^2+be1*abs(I)*sign(I))/(ae0+ae1*Z+ae2*Z^2+ae3*Z^3)) + ((-1)/(as0+as1*Z+as2*Z^2+as3*Z^3));

== matlab function DYNctl_ver4_etud_Avec_AsservissementNONfonctionnel/ModeleNonLineaire1/Modele_NonLineaire/IC_to_FC/MATLAB Function ==
  data: I input; F output; Z input; ae0 parameter; ae1 parameter; ae2 parameter; ae3 parameter; as0 parameter; as1 parameter; as2 parameter; as3 parameter; be1 parameter
function F = fcn(I,Z,ae0, ae1, ae2, ae3, as0, as1, as2, as3,be1)

F = ((I^2+be1*abs(I)*sign(I))/(ae0+ae1*Z+ae2*Z^2+ae3*Z^3)) + ((-1)/(as0+as1*Z+as2*Z^2+as3*Z^3));

== matlab function DYNctl_ver4_etud_Avec_AsservissementNONfonctionnel/ModeleNonLineaire1/Modele_NonLineaire/F_to_Vz/MATLAB Function ==
  data: FA input; d2z output; FB input; g parameter; mtot parameter; FC input
function d2z = fcn(FA,FB,g,mtot, FC)

d2z = g+(FA+FB+FC)/mtot;

== matlab function DYNctl_ver4_etud_Avec_AsservissementNONfonctionnel/ModeleNonLineaire1/Modele_NonLineaire/IA_to_FA/MATLAB Function ==
  data: I input; F output; Z input; ae0 parameter; ae1 parameter; ae2 parameter; ae3 parameter; as0 parameter; as1 parameter; as2 parameter; as3 parameter; be1 parameter
function F = fcn(I,Z,ae0, ae1, ae2, ae3, as0, as1, as2, as3,be1)

F = ((I^2+be1*abs(I)*sign(I))/(ae0+ae1*Z+ae2*Z^2+ae3*Z^3)) + ((-1)/(as0+as1*Z+as2*Z^2+as3*Z^3));

== matlab function DYNctl_ver4_etud_Avec_AsservissementNONfonctionnel/ModeleNonLineaire1/Modele_NonLineaire/F_to_WxAx/MATLAB Function ==
  data: FB input; FC input; Py input; Ax input; g parameter; mS parameter; d2phi output; Jy parameter; YC parameter; YB parameter
function d2phi = fcn(FB,FC,Py,Ax,g,mS, Jy, YC, YB)

d2phi = ((FC*YC+FB*YB-(mS*g*Py))*cosd(Ax))/Jy;
